simulink model "quad"  (R2015b)
settings: Solver=VariableStepAuto  StartTime=0.0  StopTime=10.0  RelTol=1e-3
InitFcn:
  | main
values from neighbouring files (symbols this model uses):
  state0 = [0;0;0;0;0;0;0;0;0;0;0;0]    [init.m]    (also in main.m = [0;0;0;0;0;0;0;0;0.1;0;0;0])
settings Model: Creator=zhoushibo  LastModifiedBy=zhoushibo

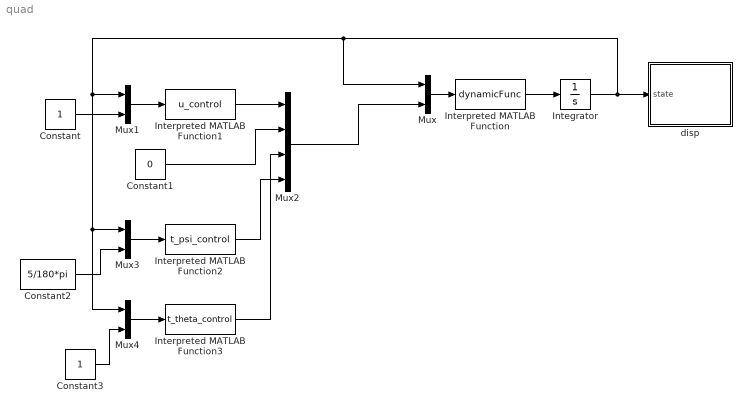
== system quad ==
  Constant : Constant
  Constant1 : Constant  Value=0
  Constant2 : Constant  Value=5/180*pi
  Constant3 : Constant
  Integrator : Integrator  InitialCondition=state0
  Interpreted MATLAB Function : MATLABFcn  MATLABFcn=dynamicFunc  OutputDimensions=12
  Interpreted MATLAB Function1 : MATLABFcn  MATLABFcn=u_control  OutputDimensions=1
  Interpreted MATLAB Function2 : MATLABFcn  MATLABFcn=t_psi_control  OutputDimensions=1
  Interpreted MATLAB Function3 : MATLABFcn  MATLABFcn=t_theta_control  OutputDimensions=1
  Mux{,1,3..4} (4 alike) : Mux  Inputs=2
  Mux2 : Mux
  disp : Subsystem
  wires:
  Interpreted MATLAB Function/1 -> Integrator/1
  Integrator/1 -> disp/1(state), Mux/1, Mux3/1, Mux4/1, Mux1/1
  Mux/1 -> Interpreted MATLAB Function/1
  Mux2/1 -> Mux/2
  Mux1/1 -> Interpreted MATLAB Function1/1
  Constant/1 -> Mux1/2
  Interpreted MATLAB Function1/1 -> Mux2/1
  Constant1/1 -> Mux2/2
  Interpreted MATLAB Function2/1 -> Mux2/4
  Mux3/1 -> Interpreted MATLAB Function2/1
  Constant2/1 -> Mux3/2
  Interpreted MATLAB Function3/1 -> Mux2/3
  Mux4/1 -> Interpreted MATLAB Function3/1
  Constant3/1 -> Mux4/2

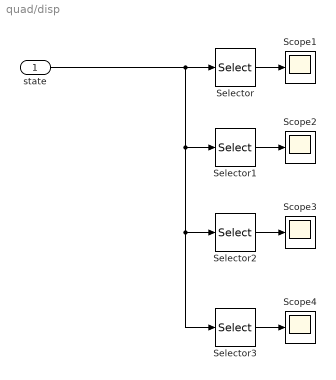
== system quad/disp ==
  state : Inport
  Scope{1..4} (4 alike) : Scope
  Selector : Selector  InputPortWidth=12  IndexOptions=Index vector (dialog)  Indices=[1:3]  OutputSizes=1
  Selector1 : Selector  InputPortWidth=12  IndexOptions=Index vector (dialog)  Indices=[4:6]  OutputSizes=1
  Selector2 : Selector  InputPortWidth=12  IndexOptions=Index vector (dialog)  Indices=[7:9]  OutputSizes=1
  Selector3 : Selector  InputPortWidth=12  IndexOptions=Index vector (dialog)  Indices=[10:12]  OutputSizes=1
  wires:
  Selector3/1 -> Scope4/1
  Selector/1 -> Scope1/1
  Selector1/1 -> Scope2/1
  Selector2/1 -> Scope3/1
  state/1 -> Selector2/1, Selector3/1, Selector1/1, Selector/1
